simulink model "Heave_NREL_solve_4cyl"  (R2020b)
settings: Solver=ode15s  StartTime=0  StopTime=200  FixedStep=0.00125  MaxStep=0.00125  RelTol=1e-3  AbsTol=1e-3  EnableMultiTasking=on
values from neighbouring files (symbols this model uses):
  simu = simulationClass()    [wecSimInputFile.m]
  waves = waveClass('irregular')    [wecSimInputFile.m]
undefined symbols (not defined in the file or in its folder): body, constraint, DiscIntNeverNeededParam, pto, X, Y, Z
libraries: fl_lib x638, nesl_utility x383, sh_lib x305, sm_lib x11, WECSim_Lib x10, fl_ps_legacy_lib x1
(part 1 of 25)
settings Model: Creator=mlawson  LastModifiedBy=mkell
settings SolverCC: AutoScaleAbsTol=off  ZeroCrossControl=DisableAll  AlgebraicLoopSolver=LineSearch  AutoInsertRateTranBlk=on
settings DataIOCC: SaveFormat=Array  SaveOutput=off  SaveTime=off  ReturnWorkspaceOutputs=off
settings OptimizationCC: LifeSpan=inf  SimCompilerOptimization=on
settings DebuggingCC: UnderspecifiedInitializationDetection=Classic  MergeDetectMultiDrivingBlocksExec=none  SolverPrmCheckMsg=warning  AllowSymbolicDim=off  StateNameClashWarn=warning  SFUnexpectedBacktrackingDiag=warning  SFNoUnconditionalDefaultTransitionDiag=warning  SFExecutionAtInitializationDiag=none  ArithmeticOperatorsInVariantConditions=warning
settings HardwareCC: ProdBitPerPointer=32  ProdBitPerSizeT=32  ProdBitPerPtrDiffT=32  ProdLargestAtomicFloat=None  ProdIntDivRoundTo=Undefined  ProdEndianess=Unspecified  ProdWordSize=32  ProdHWDeviceType=32-bit Generic
settings ModelReferenceCC: PropagateSignalLabelsOutOfModel=off
settings SFSimCC: SimUseLocalCustomCode=off  CustomCodeUndefinedFunction=UseInterfaceOnly
settings RTWCC: RTWUseLocalCustomCode=off
settings CodeAppCC: StateflowObjectComments=on
settings GRTTargetCC: TargetLangStandard=C89/C90 (ANSI)
settings ConfigComp: CovMetricSettings=dw  CovSaveCumulativeToWorkspaceVar=on  CovSaveSingleToWorkspaceVar=on  CovExternalEMLEnable=off  CovSFcnEnable=off
settings SimscapeCC: SimscapeNormalizeSystem=off  SimscapeLogType=all  SimscapeLogOpenViewer=on  SimscapeLogLimitData=off  SimscapeLogDataHistory=100000

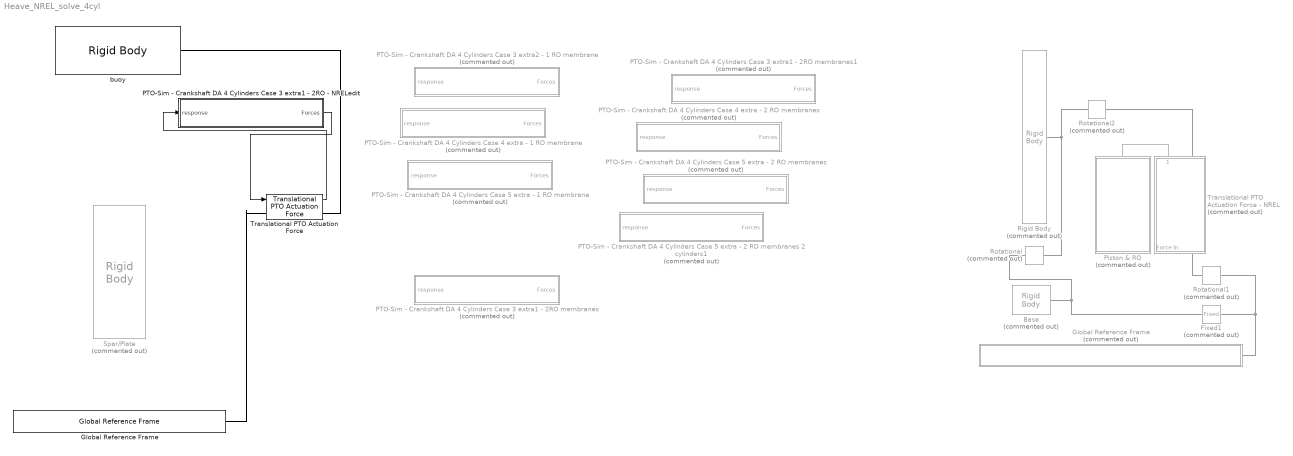
== system Heave_NREL_solve_4cyl ==
  Base : WECSim_Lib/Body Elements/Rigid Body  Commented=on  body=body(2)
      settings: AttributesFormatString=%<body>  SourceProductName=WEC-Sim
  Fixed1 : WECSim_Lib/Constraints/Fixed  Commented=on  constraint=constraint(1)
      settings: AttributesFormatString=%<constraint>  SourceProductName=WEC-Sim
  Global Reference Frame : Subsystem  Commented=on  AncestorBlock=WECSim_Lib/Frames/Global Reference Frame  mask(Frames){waves=waves, simu=simu}
      mask prompts: waves "Wave Class Name"; simu "Simulation Class Name"
      mask help:
      | This block contains Global References, including solver configurations, free surface and seabed description, and simulation time.
      | It uses the following fields from the Simulation and Wave classes:
      |
      | Simulation Class:
      |     .endTime
      |     .dt
      |     .domainSize
      |
      | Wave Class:
      |     .waterDepth
  Global Reference Frame : WECSim_Lib/Frames/Global Reference Frame  waves=waves  simu=simu
      settings: SourceProductName=WEC-Sim
  PTO-Sim - Crankshaft DA 4 Cylinders Case 3 extra1 - 2RO - NRELedit : Subsystem
  PTO-Sim - Crankshaft DA 4 Cylinders Case 3 extra1 - 2RO membranes : Subsystem  Commented=on
  PTO-Sim - Crankshaft DA 4 Cylinders Case 3 extra1 - 2RO membranes1 : Subsystem  Commented=on
  PTO-Sim - Crankshaft DA 4 Cylinders Case 3 extra2 - 1 RO membrane : Subsystem  Commented=on
  PTO-Sim - Crankshaft DA 4 Cylinders Case 4 extra - 1 RO membrane : Subsystem  Commented=on
  PTO-Sim - Crankshaft DA 4 Cylinders Case 4 extra - 2 RO membranes : Subsystem  Commented=on
  PTO-Sim - Crankshaft DA 4 Cylinders Case 5 extra - 1 RO membrane : Subsystem  Commented=on
  PTO-Sim - Crankshaft DA 4 Cylinders Case 5 extra - 2 RO membranes : Subsystem  Commented=on
  PTO-Sim - Crankshaft DA 4 Cylinders Case 5 extra - 2 RO membranes 2 cylinders1 : Subsystem  Commented=on
  "Piston & RO   " : Subsystem  Commented=on
  Rigid Body : WECSim_Lib/Body Elements/Rigid Body  Commented=on  body=body(1)
      settings: AttributesFormatString=%<body>  SourceProductName=WEC-Sim
  Rotational : WECSim_Lib/Constraints/Rotational  Commented=on  constraint=constraint(2)
      settings: AttributesFormatString=%<constraint>  SourceProductName=WEC-Sim
  Rotational1 : WECSim_Lib/Constraints/Rotational  Commented=on  constraint=constraint(3)
      settings: AttributesFormatString=%<constraint>  SourceProductName=WEC-Sim
  Rotational2 : WECSim_Lib/Constraints/Rotational  Commented=on  constraint=constraint(4)
      settings: AttributesFormatString=%<constraint>  SourceProductName=WEC-Sim
  Spar/Plate : WECSim_Lib/Body Elements/Rigid Body  Commented=on  body=body(2)
      settings: AttributesFormatString=%<body>  SourceProductName=WEC-Sim
  Translational PTO Actuation Force - NREL : Subsystem  Commented=on  AncestorBlock=WECSim_Lib/PTOs/Translational PTO Actuation Force  mask(PTO){pto=pto(1)}
      mask prompts: pto "PTO Name:"
      mask help:
      | Constraints the follower to translational motion relative to the base, in
      | the PTO's Z-direction and adds PTO stiffness and damping. Also applies a
      | user-defined force and outputs extension, velocity, and acceleration.
      |
      |
      | The variable name input below must be 'pto(i)' where i=1,2,...
      | pto(i) must be defined in the input file with the following fields:
      |
      |     .name (required)
      |             String.
      |             PTO name. Must comply with Matlab's variable naming rules.
      |     .loc (optional)
      |             3x1 vector [x y z] in meters.
      |             PTO location. Default = [0 0 0]
      |     .k (optional)
      |             Float.
      |             PTO linear spring stiffness. Default = 0
      |     .c (optional)
      |             Float.
      |             PTO linear damping coefficient. Default = 0
      |     .orientation.z (optional)
      |             3x1 vector [x y z].
      |             Direction of the PTO's Z-coordinate. Default = [0 0 1]
      |     .orientation.y (optional)
      |             3x1 vector [x y z].
      |             Direction of the PTO's Y-coordinate. Default = [0 1 0]
      mask init:
      | if exist('pto','var')
      |     h=[gcb '/output'];
      |     responseName=['pto' num2str(pto.ptoNum) '_out'];
      |     set_param(h,'VariableName',responseName);
      | end
      | 
      | pto.checkLoc('W');
      settings: AttributesFormatString=%<pto>
      mask Help:
      | Constraints the follower to translational motion relative to the base, in
      | the PTO's Z-direction and adds PTO stiffness and damping. Also applies a
      | user-defined force and outputs extension, velocity, and acceleration.
      | 
      | 
      | The variable name input below must be 'pto(i)' where i=1,2,...
      | pto(i) must be defined in the input file with the following fields:
      | 
      |     .name (required)
      |             String.
      |             PTO name. Must comply with Matlab's variable naming rules.
      |     .loc (optional)
      |             3x1 vector [x y z] in meters.
      |             PTO location. Default = [0 0 0]
      |     .k (optional)
      |             Float.
      |             PTO linear spring stiffness. Default = 0
      |     .c (optional)
      |             Float.
      |             PTO linear damping coefficient. Default = 0
      |     .orientation.z (optional)
      |             3x1 vector [x y z].
      |             Direction of the PTO's Z-coordinate. Default = [0 0 1]
      |     .orientation.y (optional)
      |             3x1 vector [x y z].
      |             Direction of the PTO's Y-coordinate. Default = [0 1 0]
  Translational PTO Actuation Force : WECSim_Lib/PTOs/Translational PTO Actuation Force  pto=pto(1)
      settings: AttributesFormatString=%<pto>  SourceProductName=WEC-Sim
  buoy : WECSim_Lib/Body Elements/Rigid Body  body=body(1)
      settings: AttributesFormatString=%<body>  SourceProductName=WEC-Sim
  wires:
  ? -> Translational PTO Actuation Force - NREL/1(Force In)
  Translational PTO Actuation Force - NREL/1(Velocity Out) -> ?
  Translational PTO Actuation Force/1 -> PTO-Sim - Crankshaft DA 4 Cylinders Case 3 extra1 - 2RO - NRELedit/1(response)
  PTO-Sim - Crankshaft DA 4 Cylinders Case 3 extra1 - 2RO - NRELedit/1(Forces) -> Translational PTO Actuation Force/1
  connections:
  Fixed1/LConn1 -- Rotational1/LConn1 -- Global Reference Frame/RConn1
  Fixed1/RConn1 -- Rotational/LConn1 -- Base/RConn1
  Rotational2/RConn1 -- Rigid Body/RConn1 -- Rotational/RConn1
  Rotational1/RConn1 -- Translational PTO Actuation Force - NREL/LConn1
  Rotational2/LConn1 -- Translational PTO Actuation Force - NREL/RConn1
  buoy/RConn1 -- Translational PTO Actuation Force/RConn1
  Global Reference Frame/RConn1 -- Translational PTO Actuation Force/LConn1

== system Heave_NREL_solve_4cyl/Global Reference Frame ==
  Clock : Clock
  Mean Free Surface : sm_lib/Body Elements/Extruded Solid  GraphicAmbientColor=[0.15 0.15 0.15 1.0]  BasedOnType=Density  CenterOfMass=[0 0 0]  CenterOfMassUnits=m  GraphicDiffuseColor=[0.0 0.6 0.8]  ExportConvexHullGeometry=off  ExtrusionCrossSection=[simu.domainSize simu.domainSize; -simu.domainSize simu.domainSize; -simu.domainSize -simu.domainSize; simu.domainSize -simu.domainSize]  ExtrusionCrossSectionUnits=m  Density=1000  DensityUnits=kg/(m^3)  DoExposeReferenceFrame=on  GraphicEmissiveColor=[0.0 0.0 0.0 1.0]  ExportEntireGeometry=off  ExtrusionLength=simu.domainSize/200  ExtrusionLengthUnits=m  ExtrusionType=General  SerializedFrames=<Frames/>  MarkerShape=Sphere  MarkerSize=10  GraphicType=FromGeometry  InertiaType=Custom  Mass=10^20  MassUnits=kg  MomentsOfInertia=[10^20 10^20 10^20]  MomentsOfInertiaUnits=kg*m^2  PolygonNumSides=3  GraphicOpacity=0.3  PolygonOuterRadius=1  PolygonOuterRadiusUnits=m  ProductsOfInertia=[0 0 0]  ProductsOfInertiaUnits=kg*m^2  GraphicShininess=75  GraphicSpecularColor=[0.5 0.5 0.5 1.0]  GraphicVisPropType=SimpleVisualProperties
  Mechanism Configuration : sm_lib/Utilities/Mechanism Configuration  UniformGravity=Constant  GravityVector=[0 0 0]  GravityVectorUnits=m/s^2  GravityUnits=m/s^2  LinearizationDelta=0.001  JointModeTransitionNonlinearIterations=2
  Rigid Transform : sm_lib/Frames and Transforms/Rigid Transform  TranslationMethod=Cartesian  TranslationStandardOffset=0  TranslationLengthUnit=m  TranslationStandardAxis=+Z  TranslationCartesianOffset=[0 0 -waves.waterDepth]  TranslationROffset=0  TranslationROffsetUnits=m  TranslationZOffset=0  TranslationZOffsetUnits=m  TranslationThetaOffset=0  TranslationThetaOffsetUnits=deg  RotationMethod=None  RotationAngleUnits=deg  RotationStandardAxis=+Z  RotationAngle=0  RotationArbitraryAxis=[0 0 1]  FollAlignAxisA=+X  BaseAlignAxisA=+Y  FollAlignAxisB=+Y  BaseAlignAxisB=+Z  RotationSequenceAxes=FollowerAxes  RotationSequence=XYX  RotationSequenceAngles=[0 0 0]  RotationSequenceAnglesUnits=deg  RotationMatrix=[1 0 0; 0 1 0; 0 0 1]
  Seabed : sm_lib/Body Elements/Extruded Solid  GraphicAmbientColor=[0.15 0.15 0.15 1.0]  BasedOnType=Density  CenterOfMass=[0 0 0]  CenterOfMassUnits=m  GraphicDiffuseColor=[0.4 0.4 0.0]  ExportConvexHullGeometry=off  ExtrusionCrossSection=[simu.domainSize simu.domainSize; -simu.domainSize simu.domainSize; -simu.domainSize -simu.domainSize; simu.domainSize -simu.domainSize]  ExtrusionCrossSectionUnits=m  Density=1000  DensityUnits=kg/(m^3)  DoExposeReferenceFrame=on  GraphicEmissiveColor=[0.0 0.0 0.0 1.0]  ExportEntireGeometry=off  ExtrusionLength=simu.domainSize/100  ExtrusionLengthUnits=m  ExtrusionType=General  SerializedFrames=<Frames/>  MarkerShape=Sphere  MarkerSize=10  GraphicType=FromGeometry  InertiaType=Custom  Mass=10^20  MassUnits=kg  MomentsOfInertia=[10^20 10^20 10^20]  MomentsOfInertiaUnits=kg*m^2  PolygonNumSides=3  GraphicOpacity=1  PolygonOuterRadius=1  PolygonOuterRadiusUnits=m  ProductsOfInertia=[0 0 0]  ProductsOfInertiaUnits=kg*m^2  GraphicShininess=75  GraphicSpecularColor=[0.5 0.5 0.5 1.0]  GraphicVisPropType=SimpleVisualProperties
  Solver Configuration : nesl_utility/Solver Configuration  PhysicalDomain=network_engine_domain  SubClassName=solver  LeftPortType=input  RightPortType=generic  Tones=[]  Harmonics=[]  SimulateNoise=off  Profile=off  UseLocalSampling=off  EnableSwitchedLinearOptims=on  FrequencyDomain=off  UseCCode=off  RelTol=0.001  AbsTol=1e-06  MinStep=1e-09  ToWorkspace=off  RevertToSquareIcSolve=off  NumHomotopyIterations=100  PhasorMode=off  PhasorModeNumHarmonics=1  DoDC=on  ResidualTolerance=1e-9  UseLocalSolver=off  LocalSolverChoice=NE_BACKWARD_EULER_ADVANCER  LocalSolverSampleTime=0.01  DoFixedCost=off  MaxNonlinIter=3  MaxModeIter=2  ComputeImpulses=off  ImpulseIterations=2  LinearAlgebra=Sparse  EquationFormulation=NE_TIME_EF  DelaysMemoryBudget=1024  AutomaticFiltering=on  FilteringTimeConstant=0.001  PartitionStorageMethod=AS_NEEDED  PartitionMemoryBudget=1024  PartitionMethod=FAST
  World Frame : sm_lib/Frames and Transforms/World Frame
  Conn : PMIOPort  Side=Right
  tag scope: Clock=global
  wires:
  Clock/1 -> [Clock]
  connections:
  Seabed/RConn1 -- Rigid Transform/RConn1
  Rigid Transform/LConn1 -- Mean Free Surface/RConn1 -- Conn/RConn1 -- Solver Configuration/RConn1 -- World Frame/RConn1 -- Mechanism Configuration/RConn1

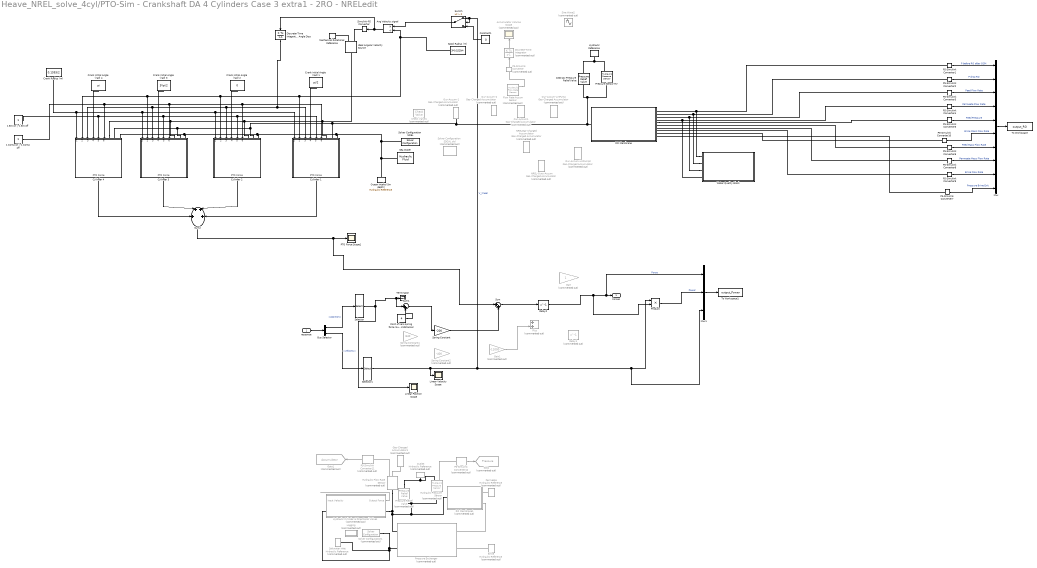
== system Heave_NREL_solve_4cyl/PTO-Sim - Crankshaft DA 4 Cylinders Case 3 extra1 - 2RO - NRELedit ==
  response : Inport
  " Flow Rate Accum Sensor" : fl_lib/Hydraulic/Hydraulic Sensors/Hydraulic Flow Rate Sensor  Commented=on
  1 Comp on | -1 Comp off : Constant
  1 Ext on | -1 Ext off : Constant
  1000 psi Pressure Relief Valve : sh_lib/Valves/Pressure Control Valves/Pressure Relief Valve  valve_area_spec=1  p_diff_TLU=[30.15e5 : 15e3 : 31.35e5] Pa  area_TLU=[1 : 1 : 9] .* 1e-5 m^2  area_max=pi*(0.75/2)^2 in^2  pres_set=1000 psi  reg_range=50 psi  C_d=0.7  A_leak=1e-12 m^2  lam_spec=1  B_lam=0.999  Re_cr=12  dynamic=0  tau=0.1 s  area_init=1e-12 m^2
      settings: SourceProductBaseCode=SH  InternalSimscapePortConfiguration="{\"Bottom\":[],\"Left\":[{\"id\":\"A\",\"label\":\"A\",\"type\":\"foundation.hydraulic.hydraulic\"}],\"Right\":[{\"id\":\"B\",\"label\":\"B\",\"type\":\"foundation.hydraulic.hydraulic\"}],\"Top\":[]}"
  Accumulator Volume Scope : Scope  Commented=on
  Ang Velocity signal : Product  Inputs=*/
  "Brine " : fl_lib/Hydraulic/Hydraulic Elements/Hydraulic Reference  Commented=on
  Bus Selector : BusSelector  OutputSignals=position,velocity
  Check Valve1 : sh_lib/Valves/Directional Valves/Check Valve  Commented=on  area_max=pi*(0.75/2)^12 in^2  pres_crack=1 psi  pres_max=4000 psi  C_d=0.7  A_leak=1e-12 m^2  lam_spec=1  B_lam=0.999  Re_cr=12  dynamic=0  tau=0.1 s  area_init=1e-12 m^2
      settings: SourceProductBaseCode=SH  InternalSimscapePortConfiguration="{\"Bottom\":[],\"Left\":[{\"id\":\"A\",\"label\":\"A\",\"type\":\"foundation.hydraulic.hydraulic\"}],\"Right\":[{\"id\":\"B\",\"label\":\"B\",\"type\":\"foundation.hydraulic.hydraulic\"}],\"Top\":[]}"
  Constant1 : Constant  Value=0
  Crank Initial Angle (rad) 1 : Constant  Value=pi/2
  Crank Initial Angle (rad) 2 : Constant  Value=0
  Crank Initial Angle (rad) 3 : Constant  Value=3*pi/2
  Crank Initial Angle (rad) 4 : Constant  Value=pi
  Crank Radius (m) : Constant  Value=0.1593/2
  Cylinder 1 : Subsystem
  Cylinder 2 : Subsystem
  Cylinder 3 : Subsystem
  Cylinder 4 : Subsystem
  Delay1 : Delay  Commented=on  DelayLength=1
  Delay2 : Delay  DelayLength=1
  Discrete-Time Integrator : DiscreteIntegrator  Commented=on  SampleTime=-1  ICPrevOutput=DiscIntNeverNeededParam  ICPrevScaledInput=DiscIntNeverNeededParam
  Discrete-Time Integrator - Angle Disp : DiscreteIntegrator  SampleTime=-1  ICPrevOutput=DiscIntNeverNeededParam  ICPrevScaledInput=DiscIntNeverNeededParam
  Gain : Gain  Commented=on
  Gain1 : Gain  Commented=on  Gain=-11000
  Gas-Charged Accumulator1 : sh_lib/Accumulators/Gas-Charged Accumulator  Commented=on  capacity=4 m^3  dead_volume=4e-5 m^3  pr_preload=30e5 Pa  k_sh=1.4  stiff_coeff=1e7 Pa/m^3  penetr_coeff=1e7 s*Pa/m^6  flow_rate_specify=off  flow_rate_priority=None  flow_rate=0 m^3/s  flow_rate_nominal_specify=off  flow_rate_nominal_unit=m^3/s  flow_rate_nominal_value=1  liquid_volume_specify=on  liquid_volume_priority=High  liquid_volume=0 m^3  liquid_volume_nominal_specify=off  liquid_volume_nominal_unit=m^3  liquid_volume_nominal_value=1  liquid_pressure_specify=off  liquid_pressure_priority=None  liquid_pressure=1.01325e+5 Pa  liquid_pressure_nominal_specify=off  liquid_pressure_nominal_unit=Pa  liquid_pressure_nominal_value=1
      settings: SourceProductBaseCode=SH  InternalSimscapePortConfiguration="{\"Bottom\":[],\"Left\":[],\"Right\":[{\"id\":\"A\",\"label\":\"A\",\"type\":\"foundation.hydraulic.hydraulic\"}],\"Top\":[]}"
  Goto : Goto  Commented=on  GotoTag=Pressure  TagVisibility=global
  Goto1 : Goto  Commented=on  GotoTag=Accumulator  TagVisibility=global
  Hydraulic Flow Rate Sensor : fl_lib/Hydraulic/Hydraulic Sensors/Hydraulic Flow Rate Sensor  Commented=on
  Hydraulic Cylinder & Directional Valves : Subsystem  Commented=on
      mask Display: image('/Users/yyu/Dropbox/WorksNREL/ResearchWork/Desalination/JSME Runs/Images/HydraulicCylinder.png');
  Hydraulic Pressure Sensor : fl_lib/Hydraulic/Hydraulic Sensors/Hydraulic Pressure Sensor  Commented=on
  Hydraulic Reference : fl_lib/Hydraulic/Hydraulic Elements/Hydraulic Reference
  Ideal Angular Velocity Source : fl_lib/Mechanical/Mechanical Sources/Ideal Angular Velocity Source
  Linear Position Scope : Scope
  Linear Velocity Scope : Scope
  Logging : Subsystem  Commented=on
  Mechanical Rotational Reference : fl_lib/Mechanical/Rotational Elements/Mechanical Rotational Reference
  Mux : Mux  Inputs=10
  Mux1 : Mux  Inputs=3
  NREL-Ours-Accum : sh_lib/Accumulators/Gas-Charged Accumulator  Commented=on  capacity=2.5 gal  dead_volume=0.04 l  pr_preload=30e5 Pa  k_sh=1.4  stiff_coeff=1e7 Pa/m^3  penetr_coeff=1e7 s*Pa/m^6  flow_rate_specify=off  flow_rate_priority=None  flow_rate=0 m^3/s  flow_rate_nominal_specify=off  flow_rate_nominal_unit=m^3/s  flow_rate_nominal_value=1  liquid_volume_specify=on  liquid_volume_priority=High  liquid_volume=0 m^3  liquid_volume_nominal_specify=off  liquid_volume_nominal_unit=m^3  liquid_volume_nominal_value=1  liquid_pressure_specify=off  liquid_pressure_priority=None  liquid_pressure=1.01325e+5 Pa  liquid_pressure_nominal_specify=off  liquid_pressure_nominal_unit=Pa  liquid_pressure_nominal_value=1
      settings: SourceProductBaseCode=SH  InternalSimscapePortConfiguration="{\"Bottom\":[],\"Left\":[],\"Right\":[{\"id\":\"A\",\"label\":\"A\",\"type\":\"foundation.hydraulic.hydraulic\"}],\"Top\":[]}"
  NRELGas-Charged Accumulator : sh_lib/Accumulators/Gas-Charged Accumulator  Commented=on  capacity=4 m^3  dead_volume=4e-5 m^3  pr_preload=30e5 Pa  k_sh=1.4  stiff_coeff=1e7 Pa/m^3  penetr_coeff=1e7 s*Pa/m^6  flow_rate_specify=off  flow_rate_priority=None  flow_rate=0 m^3/s  flow_rate_nominal_specify=off  flow_rate_nominal_unit=m^3/s  flow_rate_nominal_value=1  liquid_volume_specify=on  liquid_volume_priority=High  liquid_volume=0 m^3  liquid_volume_nominal_specify=off  liquid_volume_nominal_unit=m^3  liquid_volume_nominal_value=1  liquid_pressure_specify=off  liquid_pressure_priority=None  liquid_pressure=1.01325e+5 Pa  liquid_pressure_nominal_specify=off  liquid_pressure_nominal_unit=Pa  liquid_pressure_nominal_value=1
      settings: SourceProductBaseCode=SH  InternalSimscapePortConfiguration="{\"Bottom\":[],\"Left\":[],\"Right\":[{\"id\":\"A\",\"label\":\"A\",\"type\":\"foundation.hydraulic.hydraulic\"}],\"Top\":[]}"
  Ocean Intake (5m depth) : fl_lib/Hydraulic/Hydraulic Elements/Hydraulic Reference
  Our-Accum-1 : sh_lib/Accumulators/Gas-Charged Accumulator  Commented=on  capacity=accumulator_volume l  dead_volume=minimum_gas_volume l  pr_preload=precharge_pressure Pa  k_sh=1.4  stiff_coeff=1e7 Pa/m^3  penetr_coeff=1e7 s*Pa/m^6  flow_rate_specify=on  flow_rate_priority=None  flow_rate=0 m^3/s  flow_rate_nominal_specify=off  flow_rate_nominal_unit=m^3/s  flow_rate_nominal_value=1  liquid_volume_specify=on  liquid_volume_priority=High  liquid_volume=init_accum_volume l  liquid_volume_nominal_specify=off  liquid_volume_nominal_unit=m^3  liquid_volume_nominal_value=1  liquid_pressure_specify=off  liquid_pressure_priority=None  liquid_pressure=1.01325e+5 Pa  liquid_pressure_nominal_specify=off  liquid_pressure_nominal_unit=Pa  liquid_pressure_nominal_value=1
      settings: SourceProductBaseCode=SH  InternalSimscapePortConfiguration="{\"Bottom\":[],\"Left\":[],\"Right\":[{\"id\":\"A\",\"label\":\"A\",\"type\":\"foundation.hydraulic.hydraulic\"}],\"Top\":[]}"
  Our-Accum-2 : sh_lib/Accumulators/Gas-Charged Accumulator  Commented=on  capacity=accumulator_volume l  dead_volume=minimum_gas_volume l  pr_preload=30e5 Pa  k_sh=1.4  stiff_coeff=1e7 Pa/m^3  penetr_coeff=1e7 s*Pa/m^6  flow_rate_specify=on  flow_rate_priority=None  flow_rate=0 m^3/s  flow_rate_nominal_specify=off  flow_rate_nominal_unit=m^3/s  flow_rate_nominal_value=1  liquid_volume_specify=on  liquid_volume_priority=High  liquid_volume=0 m^3  liquid_volume_nominal_specify=off  liquid_volume_nominal_unit=m^3  liquid_volume_nominal_value=1  liquid_pressure_specify=off  liquid_pressure_priority=None  liquid_pressure=1.01325e+5 Pa  liquid_pressure_nominal_specify=off  liquid_pressure_nominal_unit=Pa  liquid_pressure_nominal_value=1
      settings: SourceProductBaseCode=SH  InternalSimscapePortConfiguration="{\"Bottom\":[],\"Left\":[],\"Right\":[{\"id\":\"A\",\"label\":\"A\",\"type\":\"foundation.hydraulic.hydraulic\"}],\"Top\":[]}"
  Our-Accum-LinPump : sh_lib/Accumulators/Gas-Charged Accumulator  Commented=on  capacity=accumulator_volume l  dead_volume=minimum_gas_volume l  pr_preload=precharge_pressure Pa  k_sh=1.4  stiff_coeff=1e12 Pa/m^3  penetr_coeff=1e10 s*Pa/m^6  flow_rate_specify=off  flow_rate_priority=High  flow_rate=0 m^3/s  flow_rate_nominal_specify=off  flow_rate_nominal_unit=m^3/s  flow_rate_nominal_value=1  liquid_volume_specify=off  liquid_volume_priority=High  liquid_volume=10*5e-3 gal  liquid_volume_nominal_specify=off  liquid_volume_nominal_unit=m^3  liquid_volume_nominal_value=1  liquid_pressure_specify=off  liquid_pressure_priority=None  liquid_pressure=0 Pa  liquid_pressure_nominal_specify=off  liquid_pressure_nominal_unit=Pa  liquid_pressure_nominal_value=1
      settings: SourceProductBaseCode=SH  InternalSimscapePortConfiguration="{\"Bottom\":[],\"Left\":[],\"Right\":[{\"id\":\"A\",\"label\":\"A\",\"type\":\"foundation.hydraulic.hydraulic\"}],\"Top\":[]}"
  Our-Accum-LinPump2 : sh_lib/Accumulators/Gas-Charged Accumulator  Commented=on  capacity=accumulator_volume l  dead_volume=minimum_gas_volume l  pr_preload=precharge_pressure Pa  k_sh=1.4  stiff_coeff=1e12 Pa/m^3  penetr_coeff=1e10 s*Pa/m^6  flow_rate_specify=off  flow_rate_priority=High  flow_rate=0 m^3/s  flow_rate_nominal_specify=off  flow_rate_nominal_unit=m^3/s  flow_rate_nominal_value=1  liquid_volume_specify=off  liquid_volume_priority=High  liquid_volume=10*5e-3 gal  liquid_volume_nominal_specify=off  liquid_volume_nominal_unit=m^3  liquid_volume_nominal_value=1  liquid_pressure_specify=off  liquid_pressure_priority=None  liquid_pressure=0 Pa  liquid_pressure_nominal_specify=off  liquid_pressure_nominal_unit=Pa  liquid_pressure_nominal_value=1
      settings: SourceProductBaseCode=SH  InternalSimscapePortConfiguration="{\"Bottom\":[],\"Left\":[],\"Right\":[{\"id\":\"A\",\"label\":\"A\",\"type\":\"foundation.hydraulic.hydraulic\"}],\"Top\":[]}"
  Our-Accum1 : sh_lib/Accumulators/Gas-Charged Accumulator  Commented=on  capacity=accumulator_volume l  dead_volume=minimum_gas_volume l  pr_preload=precharge_pressure Pa  k_sh=1.4  stiff_coeff=1e12 Pa/m^3  penetr_coeff=1e10 s*Pa/m^6  flow_rate_specify=off  flow_rate_priority=High  flow_rate=0 m^3/s  flow_rate_nominal_specify=off  flow_rate_nominal_unit=m^3/s  flow_rate_nominal_value=1  liquid_volume_specify=off  liquid_volume_priority=High  liquid_volume=10*5e-3 gal  liquid_volume_nominal_specify=off  liquid_volume_nominal_unit=m^3  liquid_volume_nominal_value=1  liquid_pressure_specify=off  liquid_pressure_priority=None  liquid_pressure=0 Pa  liquid_pressure_nominal_specify=off  liquid_pressure_nominal_unit=Pa  liquid_pressure_nominal_value=1
      settings: SourceProductBaseCode=SH  InternalSimscapePortConfiguration="{\"Bottom\":[],\"Left\":[],\"Right\":[{\"id\":\"A\",\"label\":\"A\",\"type\":\"foundation.hydraulic.hydraulic\"}],\"Top\":[]}"
  Outlet : fl_lib/Hydraulic/Hydraulic Elements/Hydraulic Reference  Commented=on
  PS-Simulink Converter : nesl_utility/PS-Simulink Converter  Commented=on  PhysicalDomain=network_engine_domain  SubClassName=ps_output  LeftPortType=input  RightPortType=output  PseudoPeriodic=off  Frequencies=[]  Unit=inherit  AffineConversion=off
  PS-Simulink Converter{1..10} (10 alike) : nesl_utility/PS-Simulink Converter  PhysicalDomain=network_engine_domain  SubClassName=ps_output  LeftPortType=input  RightPortType=output  PseudoPeriodic=off  Frequencies=[]  Unit=inherit  AffineConversion=off
  PS-Simulink Converter11 : nesl_utility/PS-Simulink Converter  Commented=on  PhysicalDomain=network_engine_domain  SubClassName=ps_output  LeftPortType=input  RightPortType=output  PseudoPeriodic=off  Frequencies=[]  Unit=1  AffineConversion=off
  PS-Simulink Converter12 : nesl_utility/PS-Simulink Converter  Commented=on  PhysicalDomain=network_engine_domain  SubClassName=ps_output  LeftPortType=input  RightPortType=output  PseudoPeriodic=off  Frequencies=[]  Unit=1  AffineConversion=off
  PTO Force Scope1 : Scope
  Permeate : fl_lib/Hydraulic/Hydraulic Elements/Hydraulic Reference  Commented=on
  Plus : Sum  Commented=on
  "Point of zero spring force (submerged distance) " : Constant  Value=4
  Pressure Relief Valve : sh_lib/Valves/Pressure Control Valves/Pressure Relief Valve  Commented=on  valve_area_spec=1  p_diff_TLU=[30.15e5 : 15e3 : 31.35e5] Pa  area_TLU=[1 : 1 : 9] .* 1e-5 m^2  area_max=2.67e-2 m^2  pres_set=56e5 Pa  reg_range=1e5 Pa  C_d=0.7  A_leak=1e-12 m^2  lam_spec=1  B_lam=0.999  Re_cr=12  dynamic=1  tau=0.1 s  area_init=1e-12 m^2
      settings: SourceProductBaseCode=SH  InternalSimscapePortConfiguration="{\"Bottom\":[],\"Left\":[{\"id\":\"A\",\"label\":\"A\",\"type\":\"foundation.hydraulic.hydraulic\"}],\"Right\":[{\"id\":\"B\",\"label\":\"B\",\"type\":\"foundation.hydraulic.hydraulic\"}],\"Top\":[]}"
  Pressure Sensor RV : fl_lib/Hydraulic/Hydraulic Sensors/Hydraulic Pressure Sensor
  Pressure Exchanger : Subsystem  Commented=on
      mask Display: image('/Users/yyu/Dropbox/WorksNREL/ResearchWork/Desalination/JSME Runs/Images/PressureExchanger.png');
  Product : Product
  RO Membrane : Subsystem
  RO Membrane1 : Subsystem  Commented=on
      mask Display: image('/Users/yyu/Dropbox/WorksNREL/ResearchWork/Desalination/JSME Runs/Images/ReverseOsmosisMembrane.jpg');
  Saltwater Inlet : fl_lib/Hydraulic/Hydraulic Elements/Hydraulic Reference  Commented=on
  Sea Water : sh_lib/Hydraulic Utilities/Hydraulic Fluid  DataSource=1  SelFluid=24  SysTemp=30  TrapAir=0.005  ViscDerFactor=1  range_error=2
  Selector : Selector  InputPortWidth=6  IndexOptions=Index vector (dialog)  Indices=3  OutputSizes=1
  Selector1 : Selector  InputPortWidth=6  IndexOptions=Index vector (dialog)  Indices=3  OutputSizes=1
  Simulink-PS Converter : nesl_utility/Simulink-PS Converter  PhysicalDomain=network_engine_domain  SubClassName=ps_input  LeftPortType=input  RightPortType=output  PseudoPeriodic=off  Frequencies=[]  NoiseDistribution=none  NoiseParameters=[]  Unit=rad/s  AffineConversion=off  FilteringAndDerivatives=provide  SimscapeFilterOrder=2  InputFilterTimeConstant=0.001  UdotUserProvided=0
  Sine Wave2 : Sin  Commented=on  Amplitude=0.45/4  Frequency=0.9  SampleTime=0.01
  Solver Configuration NREL : nesl_utility/Solver Configuration  PhysicalDomain=network_engine_domain  SubClassName=solver  LeftPortType=input  RightPortType=generic  Tones=[]  Harmonics=[]  SimulateNoise=off  Profile=off  UseLocalSampling=off  EnableSwitchedLinearOptims=on  FrequencyDomain=off  UseCCode=off  RelTol=0.001  AbsTol=1e-06  MinStep=1e-09  ToWorkspace=off  RevertToSquareIcSolve=off  NumHomotopyIterations=100  PhasorMode=off  PhasorModeNumHarmonics=1  DoDC=on  ResidualTolerance=1e-09  UseLocalSolver=on  LocalSolverChoice=NE_BACKWARD_EULER_ADVANCER  LocalSolverSampleTime=simu.dt  DoFixedCost=on  MaxNonlinIter=3  MaxModeIter=2  ComputeImpulses=off  ImpulseIterations=2  LinearAlgebra=Sparse  EquationFormulation=NE_TIME_EF  DelaysMemoryBudget=1024  AutomaticFiltering=on  FilteringTimeConstant=0.001  PartitionStorageMethod=AS_NEEDED  PartitionMemoryBudget=1024  PartitionMethod=FAST
  Solver Configuration SDCAL old : nesl_utility/Solver Configuration  Commented=on  PhysicalDomain=network_engine_domain  SubClassName=solver  LeftPortType=input  RightPortType=generic  Tones=[]  Harmonics=[]  SimulateNoise=off  Profile=off  UseLocalSampling=off  EnableSwitchedLinearOptims=on  FrequencyDomain=off  UseCCode=off  RelTol=0.001  AbsTol=1e-06  MinStep=1e-09  ToWorkspace=off  RevertToSquareIcSolve=off  NumHomotopyIterations=100  PhasorMode=off  PhasorModeNumHarmonics=1  DoDC=off  ResidualTolerance=1e-09  UseLocalSolver=off  LocalSolverChoice=NE_BACKWARD_EULER_ADVANCER  LocalSolverSampleTime=0.001  DoFixedCost=off  MaxNonlinIter=3  MaxModeIter=2  ComputeImpulses=off  ImpulseIterations=2  LinearAlgebra=auto  EquationFormulation=NE_TIME_EF  DelaysMemoryBudget=1024  AutomaticFiltering=on  FilteringTimeConstant=0.01  PartitionStorageMethod=AS_NEEDED  PartitionMemoryBudget=1024  PartitionMethod=ROBUST
  Solver Configuration1 : nesl_utility/Solver Configuration  Commented=on  PhysicalDomain=network_engine_domain  SubClassName=solver  LeftPortType=input  RightPortType=generic  Tones=[]  Harmonics=[]  SimulateNoise=off  Profile=off  UseLocalSampling=off  EnableSwitchedLinearOptims=on  FrequencyDomain=off  UseCCode=off  RelTol=0.001  AbsTol=1e-06  MinStep=1e-09  ToWorkspace=off  RevertToSquareIcSolve=off  NumHomotopyIterations=100  PhasorMode=off  PhasorModeNumHarmonics=1  DoDC=on  ResidualTolerance=1e-09  UseLocalSolver=on  LocalSolverChoice=NE_BACKWARD_EULER_ADVANCER  LocalSolverSampleTime=simu.dt  DoFixedCost=on  MaxNonlinIter=3  MaxModeIter=2  ComputeImpulses=off  ImpulseIterations=2  LinearAlgebra=Sparse  EquationFormulation=NE_TIME_EF  DelaysMemoryBudget=1024  AutomaticFiltering=on  FilteringTimeConstant=0.001  PartitionStorageMethod=AS_NEEDED  PartitionMemoryBudget=1024  PartitionMethod=FAST
  Spool Radius (m) : Constant  Value=3*0.1520/4
  Spring Constant : Gain  Gain=-200
  Spring Constant1 : Gain  Commented=on  Gain=840
  Spring Constant2 : Gain  Commented=on  Gain=-400
  Sum : Sum  Inputs=|++
  Sum1 : Sum  Inputs=|++
  Sum2 : Sum  Inputs=4
  Switch : Switch  Criteria=u2 > Threshold
  Terminator : Terminator
  To Workspace : ToWorkspace  VariableName=output_RO  SaveFormat=Structure With Time  SampleTime=-1
  To Workspace1 : ToWorkspace  VariableName=output_Power  SaveFormat=Structure With Time  SampleTime=-1
  Water Quality Block : Subsystem
  Forces : Outport  VectorParamsAs1DForOutWhenUnconnected=off
  wires:
  Bus Selector/1 -> Selector/1  "<position>"
  Bus Selector/2 -> Selector1/1  "<velocity>"
  response/1 -> Bus Selector/1
  Selector/1 -> Linear Position Scope/1, Sum1/1, Terminator/1
  Spring Constant/1 -> Sum/2
  Gain1/1 -> Plus/2
  Sum/1 -> Delay2/1
  Selector1/1 -> Linear Velocity Scope/1, Mux1/3, Product/1, Switch/2, Switch/1  "V_linear"
  "Point of zero spring force (submerged distance) "/1 -> Sum1/2
  Sum1/1 -> Spring Constant/1
  Delay2/1 -> Product/2, Mux1/1, Forces/1  "Force"
  Mux1/1 -> To Workspace1/1
  Product/1 -> Mux1/2  "Power"
  1 Ext on | -1 Ext off/1 -> Cylinder 1/5(Ext Control Input), Cylinder 2/5(Ext Control Input), Cylinder 3/5(Ext Control Input), Cylinder 4/5(Ext Control Input)
  1 Comp on | -1 Comp off/1 -> Cylinder 1/6(Comp Control Input), Cylinder 2/6(Comp Control Input), Cylinder 3/6(Comp Control Input), Cylinder 4/6(Comp Control Input)
  Sum2/1 -> PTO Force Scope1/1, Sum/1
  PS-Simulink Converter7/1 -> Mux/10  "Pressure Brine Exit"
  Discrete-Time Integrator/1 -> Accumulator Volume Scope/1
  PS-Simulink Converter/1 -> Discrete-Time Integrator/1
  PS-Simulink Converter9/1 -> Mux/9  "Brine Flow Rate"
  PS-Simulink Converter5/1 -> Mux/5  "Feed Pressure"
  Cylinder 1/1(PTO Force) -> Sum2/4
  PS-Simulink Converter8/1 -> Mux/8  "Permeate Mass Flow Rate"
  PS-Simulink Converter10/1 -> Mux/6  "Brine Mass Flow Rate"
  PS-Simulink Converter6/1 -> Mux/7  "Feed Mass Flow Rate"
  PS-Simulink Converter4/1 -> Mux/4  "Permeate Flow Rate"
  PS-Simulink Converter1/1 -> Mux/1  "P before RO after OSM"
  Constant1/1 -> Switch/3
  Mux/1 -> To Workspace/1
  Cylinder 2/1(PTO Force) -> Sum2/3
  Crank Radius (m)/1 -> Cylinder 1/1(Crank Radius), Cylinder 2/1(Crank Radius), Cylinder 3/1(Crank Radius), Cylinder 4/1(Crank Radius)
  PS-Simulink Converter2/1 -> Mux/2  "P drop RO"
  Ang Velocity signal/1 -> Discrete-Time Integrator - Angle Disp/1, Simulink-PS Converter/1
  Spool Radius (m)/1 -> Cylinder 1/2(Spool Radius), Cylinder 4/2(Spool Radius), Cylinder 3/2(Spool Radius), Cylinder 2/2(Spool Radius), Ang Velocity signal/2
  Discrete-Time Integrator - Angle Disp/1 -> Cylinder 4/3(Angle Displacement), Cylinder 3/3(Angle Displacement), Cylinder 2/3(Angle Displacement), Cylinder 1/3(Angle Displacement)
  Cylinder 4/1(PTO Force) -> Sum2/1
  Crank Initial Angle (rad) 3/1 -> Cylinder 3/4(Crank Init Angle)
  Crank Initial Angle (rad) 2/1 -> Cylinder 2/4(Crank Init Angle)
  Crank Initial Angle (rad) 1/1 -> Cylinder 1/4(Crank Init Angle)
  Cylinder 3/1(PTO Force) -> Sum2/2
  Switch/1 -> Ang Velocity signal/1
  Crank Initial Angle (rad) 4/1 -> Cylinder 4/4(Crank Init Angle)
  PS-Simulink Converter3/1 -> Mux/3  "Feed Flow Rate"
  PS-Simulink Converter12/1 -> Goto/1
  PS-Simulink Converter11/1 -> Goto1/1
  Hydraulic Cylinder & Directional Valves/1(Output Force) -> ?
  connections:
  Hydraulic Reference/LConn1 -- 1000 psi Pressure Relief Valve/RConn1 -- Pressure Sensor RV/RConn1
  Water Quality Block/LConn4 -- RO Membrane/RConn4 -- PS-Simulink Converter4/LConn1
  Water Quality Block/LConn1 -- PS-Simulink Converter1/LConn1 -- RO Membrane/RConn1
  Cylinder 4/LConn1 -- Cylinder 3/LConn1 -- Cylinder 1/LConn1 -- Ideal Angular Velocity Source/LConn1 -- Cylinder 2/LConn1
  Water Quality Block/LConn3 -- PS-Simulink Converter3/LConn1 -- RO Membrane/RConn3
  Cylinder 1/LConn3 -- Solver Configuration NREL/RConn1 -- Ocean Intake (5m depth)/LConn1 -- Sea Water/RConn1 -- Cylinder 4/LConn3 -- Cylinder 3/LConn3 -- Cylinder 2/LConn3
  Water Quality Block/LConn2 -- PS-Simulink Converter2/LConn1 -- RO Membrane/RConn2
  PS-Simulink Converter10/LConn1 -- RO Membrane/RConn9
  PS-Simulink Converter8/LConn1 -- RO Membrane/RConn7
  PS-Simulink Converter7/LConn1 -- RO Membrane/RConn10
  RO Membrane/RConn5 -- PS-Simulink Converter5/LConn1
  Ideal Angular Velocity Source/RConn1 -- Simulink-PS Converter/RConn1
  PS-Simulink Converter9/LConn1 -- RO Membrane/RConn8
  PS-Simulink Converter6/LConn1 -- RO Membrane/RConn6
  Ideal Angular Velocity Source/RConn2 -- Mechanical Rotational Reference/LConn1
  " Flow Rate Accum Sensor"/RConn1 -- PS-Simulink Converter/LConn1
  RO Membrane1/LConn1 -- Hydraulic Pressure Sensor/LConn1 -- Pressure Relief Valve/LConn1 -- Hydraulic Cylinder & Directional Valves/RConn1 -- Hydraulic Flow Rate Sensor/LConn1 -- Pressure Exchanger/LConn1
  Pressure Relief Valve/RConn1 -- Outlet/LConn1 -- Hydraulic Pressure Sensor/RConn1
  Saltwater Inlet/LConn1 -- Hydraulic Cylinder & Directional Valves/LConn1 -- Pressure Exchanger/LConn2 -- Solver Configuration1/RConn1
  Hydraulic Flow Rate Sensor/RConn2 -- Gas-Charged Accumulator1/RConn1
  PS-Simulink Converter12/LConn1 -- Hydraulic Pressure Sensor/RConn2
  "Brine "/LConn1 -- Pressure Exchanger/RConn2
  Permeate/LConn1 -- RO Membrane1/RConn1
  RO Membrane1/RConn2 -- Pressure Exchanger/RConn1
  Hydraulic Flow Rate Sensor/RConn1 -- PS-Simulink Converter11/LConn1
  Cylinder 1/LConn2 -- RO Membrane/LConn1 -- Pressure Sensor RV/LConn1 -- 1000 psi Pressure Relief Valve/LConn1 -- Our-Accum-1/RConn1 -- Cylinder 3/LConn2 -- Cylinder 4/LConn2 -- Cylinder 2/LConn2

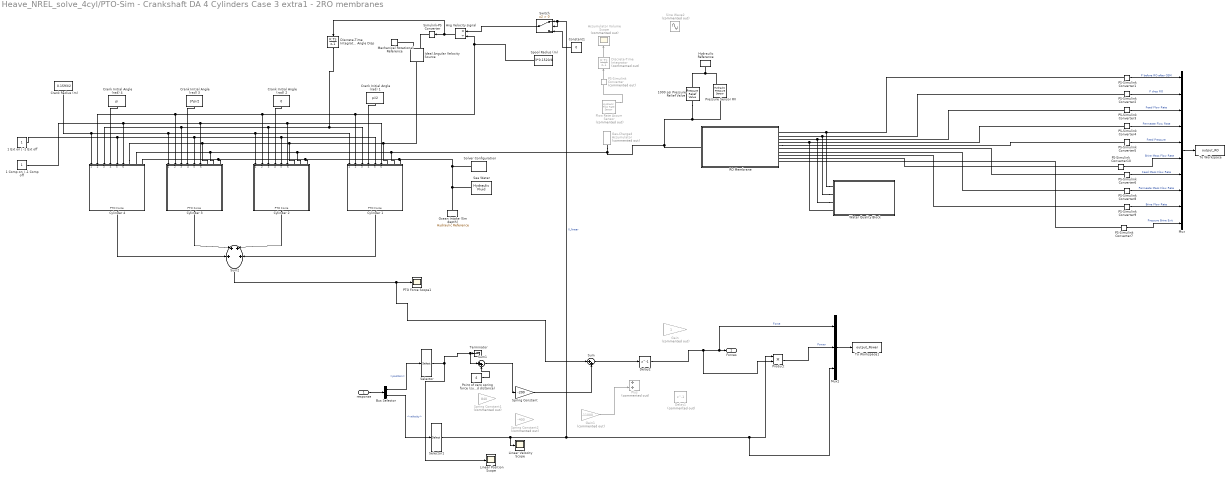
== system Heave_NREL_solve_4cyl/PTO-Sim - Crankshaft DA 4 Cylinders Case 3 extra1 - 2RO membranes ==
  response : Inport
  " Flow Rate Accum Sensor" : fl_lib/Hydraulic/Hydraulic Sensors/Hydraulic Flow Rate Sensor  Commented=on
  1 Comp on | -1 Comp off : Constant
  1 Ext on | -1 Ext off : Constant
  1000 psi Pressure Relief Valve : sh_lib/Valves/Pressure Control Valves/Pressure Relief Valve  valve_area_spec=1  p_diff_TLU=[30.15e5 : 15e3 : 31.35e5] Pa  area_TLU=[1 : 1 : 9] .* 1e-5 m^2  area_max=pi*(0.75/2)^2 in^2  pres_set=1000 psi  reg_range=50 psi  C_d=0.7  A_leak=1e-12 m^2  lam_spec=1  B_lam=0.999  Re_cr=12  dynamic=0  tau=0.1 s  area_init=1e-12 m^2
      settings: SourceProductBaseCode=SH  InternalSimscapePortConfiguration="{\"Bottom\":[],\"Left\":[{\"id\":\"A\",\"label\":\"A\",\"type\":\"foundation.hydraulic.hydraulic\"}],\"Right\":[{\"id\":\"B\",\"label\":\"B\",\"type\":\"foundation.hydraulic.hydraulic\"}],\"Top\":[]}"
  Accumulator Volume Scope : Scope  Commented=on
  Ang Velocity signal : Product  Inputs=*/
  Bus Selector : BusSelector  OutputSignals=position,velocity
  Constant1 : Constant  Value=0
  Crank Initial Angle (rad) 1 : Constant  Value=pi/2
  Crank Initial Angle (rad) 2 : Constant  Value=0
  Crank Initial Angle (rad) 3 : Constant  Value=3*pi/2
  Crank Initial Angle (rad) 4 : Constant  Value=pi
  Crank Radius (m) : Constant  Value=0.1593/2
  Cylinder 1 : Subsystem
  Cylinder 2 : Subsystem
  Cylinder 3 : Subsystem
  Cylinder 4 : Subsystem
  Delay1 : Delay  Commented=on  DelayLength=1
  Delay2 : Delay  DelayLength=1
  Discrete-Time Integrator : DiscreteIntegrator  Commented=on  SampleTime=-1  ICPrevOutput=DiscIntNeverNeededParam  ICPrevScaledInput=DiscIntNeverNeededParam
  Discrete-Time Integrator - Angle Disp : DiscreteIntegrator  SampleTime=-1  ICPrevOutput=DiscIntNeverNeededParam  ICPrevScaledInput=DiscIntNeverNeededParam
  Gain : Gain  Commented=on
  Gain1 : Gain  Commented=on  Gain=-11000
  Gas-Charged Accumulator : sh_lib/Accumulators/Gas-Charged Accumulator  Commented=on  capacity=2.5 gal  dead_volume=4e-5 m^3  pr_preload=800 psi  k_sh=1.4  stiff_coeff=1e10 Pa/m^3  penetr_coeff=1e10 s*Pa/m^6  flow_rate_specify=off  flow_rate_priority=None  flow_rate=0.005 m^3/s  flow_rate_nominal_specify=off  flow_rate_nominal_unit=m^3/s  flow_rate_nominal_value=1  liquid_volume_specify=on  liquid_volume_priority=High  liquid_volume=0.005 m^3  liquid_volume_nominal_specify=off  liquid_volume_nominal_unit=m^3  liquid_volume_nominal_value=1  liquid_pressure_specify=off  liquid_pressure_priority=None  liquid_pressure=1.01325e+5 Pa  liquid_pressure_nominal_specify=off  liquid_pressure_nominal_unit=Pa  liquid_pressure_nominal_value=1
      settings: SourceProductBaseCode=SH  InternalSimscapePortConfiguration="{\"Bottom\":[],\"Left\":[],\"Right\":[{\"id\":\"A\",\"label\":\"A\",\"type\":\"foundation.hydraulic.hydraulic\"}],\"Top\":[]}"
  Hydraulic Reference : fl_lib/Hydraulic/Hydraulic Elements/Hydraulic Reference
  Ideal Angular Velocity Source : fl_lib/Mechanical/Mechanical Sources/Ideal Angular Velocity Source
  Linear Position Scope : Scope
  Linear Velocity Scope : Scope
  Mechanical Rotational Reference : fl_lib/Mechanical/Rotational Elements/Mechanical Rotational Reference
  Mux : Mux  Inputs=10
  Mux1 : Mux  Inputs=3
  Ocean Intake (5m depth) : fl_lib/Hydraulic/Hydraulic Elements/Hydraulic Reference
  PS-Simulink Converter : nesl_utility/PS-Simulink Converter  Commented=on  PhysicalDomain=network_engine_domain  SubClassName=ps_output  LeftPortType=input  RightPortType=output  PseudoPeriodic=off  Frequencies=[]  Unit=inherit  AffineConversion=off
  PS-Simulink Converter{1..10} (10 alike) : nesl_utility/PS-Simulink Converter  PhysicalDomain=network_engine_domain  SubClassName=ps_output  LeftPortType=input  RightPortType=output  PseudoPeriodic=off  Frequencies=[]  Unit=inherit  AffineConversion=off
  PTO Force Scope1 : Scope
  Plus : Sum  Commented=on
  "Point of zero spring force (submerged distance) " : Constant  Value=4
  Pressure Sensor RV : fl_lib/Hydraulic/Hydraulic Sensors/Hydraulic Pressure Sensor
  Product : Product
  RO Membrane : Subsystem
  Sea Water : sh_lib/Hydraulic Utilities/Hydraulic Fluid  DataSource=1  SelFluid=24  SysTemp=30  TrapAir=0.005  ViscDerFactor=1  range_error=2
  Selector : Selector  InputPortWidth=6  IndexOptions=Index vector (dialog)  Indices=3  OutputSizes=1
  Selector1 : Selector  InputPortWidth=6  IndexOptions=Index vector (dialog)  Indices=3  OutputSizes=1
  Simulink-PS Converter : nesl_utility/Simulink-PS Converter  PhysicalDomain=network_engine_domain  SubClassName=ps_input  LeftPortType=input  RightPortType=output  PseudoPeriodic=off  Frequencies=[]  NoiseDistribution=none  NoiseParameters=[]  Unit=rad/s  AffineConversion=off  FilteringAndDerivatives=filter  SimscapeFilterOrder=2  InputFilterTimeConstant=0.001  UdotUserProvided=0
  Sine Wave2 : Sin  Commented=on  Amplitude=0.45/4  Frequency=0.9  SampleTime=0.01
  Solver Configuration : nesl_utility/Solver Configuration  PhysicalDomain=network_engine_domain  SubClassName=solver  LeftPortType=input  RightPortType=generic  Tones=[]  Harmonics=[]  SimulateNoise=off  Profile=off  UseLocalSampling=off  EnableSwitchedLinearOptims=on  FrequencyDomain=off  UseCCode=off  RelTol=0.001  AbsTol=1e-06  MinStep=1e-09  ToWorkspace=off  RevertToSquareIcSolve=off  NumHomotopyIterations=100  PhasorMode=off  PhasorModeNumHarmonics=1  DoDC=off  ResidualTolerance=1e-09  UseLocalSolver=off  LocalSolverChoice=NE_BACKWARD_EULER_ADVANCER  LocalSolverSampleTime=0.001  DoFixedCost=off  MaxNonlinIter=3  MaxModeIter=2  LinearAlgebra=auto  EquationFormulation=NE_TIME_EF  DelaysMemoryBudget=1024  AutomaticFiltering=on  FilteringTimeConstant=0.01  PartitionStorageMethod=AS_NEEDED  PartitionMemoryBudget=1024  PartitionMethod=ROBUST
  Spool Radius (m) : Constant  Value=3*0.1520/4
  Spring Constant : Gain  Gain=-200
  Spring Constant1 : Gain  Commented=on  Gain=840
  Spring Constant2 : Gain  Commented=on  Gain=-400
  Sum : Sum  Inputs=|++
  Sum1 : Sum  Inputs=|++
  Sum2 : Sum  Inputs=4
  Switch : Switch  Criteria=u2 > Threshold
  Terminator : Terminator
  To Workspace : ToWorkspace  VariableName=output_RO  SaveFormat=Structure With Time  SampleTime=-1
  To Workspace1 : ToWorkspace  VariableName=output_Power  SaveFormat=Structure With Time  SampleTime=-1
  Water Quality Block : Subsystem
  Forces : Outport  VectorParamsAs1DForOutWhenUnconnected=off
  wires:
  Bus Selector/1 -> Selector/1  "<position>"
  Bus Selector/2 -> Selector1/1  "<velocity>"
  response/1 -> Bus Selector/1
  Selector/1 -> Linear Position Scope/1, Sum1/1, Terminator/1
  Spring Constant/1 -> Sum/2
  Gain1/1 -> Plus/2
  Sum/1 -> Delay2/1
  Selector1/1 -> Linear Velocity Scope/1, Mux1/3, Product/1, Switch/2, Switch/1  "V_linear"
  "Point of zero spring force (submerged distance) "/1 -> Sum1/2
  Sum1/1 -> Spring Constant/1
  Delay2/1 -> Product/2, Mux1/1, Forces/1  "Force"
  Mux1/1 -> To Workspace1/1
  Product/1 -> Mux1/2  "Power"
  1 Ext on | -1 Ext off/1 -> Cylinder 1/5(Ext Control Input), Cylinder 2/5(Ext Control Input), Cylinder 3/5(Ext Control Input), Cylinder 4/5(Ext Control Input)
  1 Comp on | -1 Comp off/1 -> Cylinder 1/6(Comp Control Input), Cylinder 2/6(Comp Control Input), Cylinder 3/6(Comp Control Input), Cylinder 4/6(Comp Control Input)
  Sum2/1 -> PTO Force Scope1/1, Sum/1
  PS-Simulink Converter7/1 -> Mux/10  "Pressure Brine Exit"
  Discrete-Time Integrator/1 -> Accumulator Volume Scope/1
  PS-Simulink Converter/1 -> Discrete-Time Integrator/1
  PS-Simulink Converter9/1 -> Mux/9  "Brine Flow Rate"
  PS-Simulink Converter5/1 -> Mux/5  "Feed Pressure"
  Cylinder 1/1(PTO Force) -> Sum2/4
  PS-Simulink Converter8/1 -> Mux/8  "Permeate Mass Flow Rate"
  PS-Simulink Converter10/1 -> Mux/6  "Brine Mass Flow Rate"
  PS-Simulink Converter6/1 -> Mux/7  "Feed Mass Flow Rate"
  PS-Simulink Converter4/1 -> Mux/4  "Permeate Flow Rate"
  PS-Simulink Converter1/1 -> Mux/1  "P before RO after OSM"
  Constant1/1 -> Switch/3
  Mux/1 -> To Workspace/1
  Cylinder 2/1(PTO Force) -> Sum2/3
  Crank Radius (m)/1 -> Cylinder 1/1(Crank Radius), Cylinder 2/1(Crank Radius), Cylinder 3/1(Crank Radius), Cylinder 4/1(Crank Radius)
  PS-Simulink Converter2/1 -> Mux/2  "P drop RO"
  Ang Velocity signal/1 -> Discrete-Time Integrator - Angle Disp/1, Simulink-PS Converter/1
  Spool Radius (m)/1 -> Cylinder 1/2(Spool Radius), Cylinder 4/2(Spool Radius), Cylinder 3/2(Spool Radius), Cylinder 2/2(Spool Radius), Ang Velocity signal/2
  Discrete-Time Integrator - Angle Disp/1 -> Cylinder 4/3(Angle Displacement), Cylinder 3/3(Angle Displacement), Cylinder 2/3(Angle Displacement), Cylinder 1/3(Angle Displacement)
  Cylinder 4/1(PTO Force) -> Sum2/1
  Crank Initial Angle (rad) 3/1 -> Cylinder 3/4(Crank Init Angle)
  Crank Initial Angle (rad) 2/1 -> Cylinder 2/4(Crank Init Angle)
  Crank Initial Angle (rad) 1/1 -> Cylinder 1/4(Crank Init Angle)
  Cylinder 3/1(PTO Force) -> Sum2/2
  Switch/1 -> Ang Velocity signal/1
  Crank Initial Angle (rad) 4/1 -> Cylinder 4/4(Crank Init Angle)
  PS-Simulink Converter3/1 -> Mux/3  "Feed Flow Rate"
  connections:
  Hydraulic Reference/LConn1 -- 1000 psi Pressure Relief Valve/RConn1 -- Pressure Sensor RV/RConn1
  Water Quality Block/LConn4 -- RO Membrane/RConn4 -- PS-Simulink Converter4/LConn1
  Water Quality Block/LConn1 -- PS-Simulink Converter1/LConn1 -- RO Membrane/RConn1
  Cylinder 4/LConn1 -- Cylinder 3/LConn1 -- Cylinder 1/LConn1 -- Ideal Angular Velocity Source/LConn1 -- Cylinder 2/LConn1
  Water Quality Block/LConn3 -- PS-Simulink Converter3/LConn1 -- RO Membrane/RConn3
  Cylinder 1/LConn3 -- Cylinder 4/LConn3 -- Cylinder 3/LConn3 -- Cylinder 2/LConn3 -- Solver Configuration/RConn1 -- Ocean Intake (5m depth)/LConn1 -- Sea Water/RConn1
  Pressure Sensor RV/LConn1 -- 1000 psi Pressure Relief Valve/LConn1 -- RO Membrane/LConn1 -- Gas-Charged Accumulator/RConn1 -- Cylinder 1/LConn2 -- Cylinder 3/LConn2 -- Cylinder 4/LConn2 -- Cylinder 2/LConn2
  Water Quality Block/LConn2 -- PS-Simulink Converter2/LConn1 -- RO Membrane/RConn2
  PS-Simulink Converter10/LConn1 -- RO Membrane/RConn9
  PS-Simulink Converter8/LConn1 -- RO Membrane/RConn7
  PS-Simulink Converter7/LConn1 -- RO Membrane/RConn10
  RO Membrane/RConn5 -- PS-Simulink Converter5/LConn1
  Ideal Angular Velocity Source/RConn1 -- Simulink-PS Converter/RConn1
  PS-Simulink Converter9/LConn1 -- RO Membrane/RConn8
  PS-Simulink Converter6/LConn1 -- RO Membrane/RConn6
  Ideal Angular Velocity Source/RConn2 -- Mechanical Rotational Reference/LConn1
  " Flow Rate Accum Sensor"/RConn1 -- PS-Simulink Converter/LConn1
